simulink model "absolute"  (R2015a)
settings: Solver=ode45  SolverMode=SingleTasking  StartTime=0.0  StopTime=10.0  RelTol=1e-3
model workspace (MAT data in the model file):
  ContractValidatorBlocksMap = containers.Map
  ContractValidatorBlocksMap.serialization.keys = {'absolute/contract/validator'}
  ContractValidatorBlocksMap.serialization.values{1}.block = 'absolute/contract/validator'
  ContractValidatorBlocksMap.serialization.values{1}.assumePorts = 0
  ContractValidatorBlocksMap.serialization.values{1}.guaranteePorts = 2
  ContractValidatorBlocksMap.serialization.values{1}.modeBlocksPorts = 0
  ContractValidatorBlocksMap.serialization.values{1}.portHandles.Inport = [62.0009765625 63.0004882812]
  ContractValidatorBlocksMap.serialization.values{1}.portHandles.Outport = 64.0004882812
  ContractValidatorBlocksMap.serialization.values{1}.portHandles.Enable = []
  ContractValidatorBlocksMap.serialization.values{1}.portHandles.Trigger = []
  ContractValidatorBlocksMap.serialization.values{1}.portHandles.State = []
  ContractValidatorBlocksMap.serialization.values{1}.portHandles.LConn = []
  ContractValidatorBlocksMap.serialization.values{1}.portHandles.RConn = []
  ContractValidatorBlocksMap.serialization.values{1}.portHandles.Ifaction = []
  ContractValidatorBlocksMap.serialization.values{1}.portHandles.Reset = []
  ContractValidatorBlocksMap.serialization.values{1}.portConnectivity(1).Type = '1'
  ContractValidatorBlocksMap.serialization.values{1}.portConnectivity(1).Position = [365 -50]
  ContractValidatorBlocksMap.serialization.values{1}.portConnectivity(1).SrcBlock = 36.0014648438
  ContractValidatorBlocksMap.serialization.values{1}.portConnectivity(1).SrcPort = 0
  ContractValidatorBlocksMap.serialization.values{1}.portConnectivity(1).DstBlock = []
  ContractValidatorBlocksMap.serialization.values{1}.portConnectivity(1).DstPort = []
  ContractValidatorBlocksMap.serialization.values{1}.portConnectivity(2).Type = '2'
  ContractValidatorBlocksMap.serialization.values{1}.portConnectivity(2).Position = [365 200]
  ContractValidatorBlocksMap.serialization.values{1}.portConnectivity(2).SrcBlock = 22.0004882812
  ContractValidatorBlocksMap.serialization.values{1}.portConnectivity(2).SrcPort = 0
  ContractValidatorBlocksMap.serialization.values{1}.portConnectivity(2).DstBlock = []
  ContractValidatorBlocksMap.serialization.values{1}.portConnectivity(2).DstPort = []
  ContractValidatorBlocksMap.serialization.values{1}.portConnectivity(3).Type = '1'
  ContractValidatorBlocksMap.serialization.values{1}.portConnectivity(3).Position = [500 75]
  ContractValidatorBlocksMap.serialization.values{1}.portConnectivity(3).SrcBlock = []
  ContractValidatorBlocksMap.serialization.values{1}.portConnectivity(3).SrcPort = []
  ContractValidatorBlocksMap.serialization.values{1}.portConnectivity(3).DstBlock = 44.0009765625
  ContractValidatorBlocksMap.serialization.values{1}.portConnectivity(3).DstPort = 0
  ContractValidatorBlocksMap.serialization.uniformity = 0
  ContractValidatorBlocksMap.serialization.keyType = 'char'
  ContractValidatorBlocksMap.serialization.valueType = 'any'
undefined symbols (not defined in the file or in its folder): contractAfterSimulation, contractBeforeSimulation, saveValidatorParameters
undefined symbols (not defined in the file): ContractBlock, ContractGuaranteeBlock, ContractValidatorBlock
libraries: simulink x2
settings Model: CovMetricSettings=dwe  CovHtmlReporting=off  covSaveCumulativeToWorkspaceVar=off  CovSaveSingleToWorkspaceVar=off  CovExternalEMLEnable=on  Creator=mahgoubyahia  LastModifiedBy=hbourbou
settings DataIOCC: LimitDataPoints=off  SaveFormat=Dataset
settings DebuggingCC: SFUnexpectedBacktrackingDiag=error  SFNoUnconditionalDefaultTransitionDiag=error
settings HardwareCC: ProdBitPerPointer=64  ProdLargestAtomicFloat=Float  ProdIntDivRoundTo=Zero  ProdEndianess=LittleEndian  ProdHWDeviceType=Specified
settings ModelReferenceCC: PropagateSignalLabelsOutOfModel=on
settings GRTTargetCC: TargetLangStandard=C99 (ISO)  GeneratePreprocessorConditionals=Use local settings

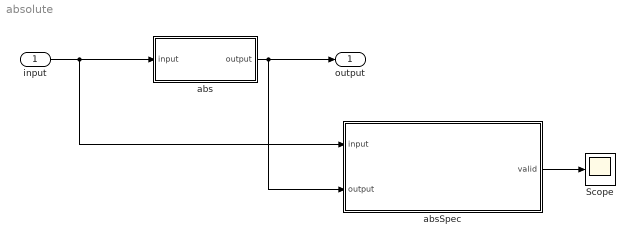
== system absolute ==
  input : Inport  OutDataTypeStr=int32
  Scope : Scope
      settings: TimeRange=auto  MaxDataPoints=5000  SaveToWorkspace=off  SaveName=ScopeData  YMin=-10  YMax=10  SampleTime=-1
  abs : Subsystem
  absSpec : Subsystem  mask{ContractBlockType=ContractBlock}
      mask init:
      | set_param(gcb, 'LinkStatus', 'none');
      mask DialogControl DescTextVar Prompt: Contract block
      mask Display:
      | text(0.5, 0.5, '{\bf\fontsize{20}Contract}', 'hor', 'center', 'texmode','on');
      | blocks = find_system(gcb, 'LookUnderMasks','all', 'SearchDepth',1,'BlockType','Inport');
      | for i = 1 : length(blocks)
      |     blockName = get_param(blocks(i), 'Name');
      |     [path, blockName] = fileparts(char(blockName));
      |     port_label('input', i, blockName);
      | end
      | 
      | blocks = find_system(gcb, 'LookUnderMasks','all', 'SearchDepth',1,'BlockType','Outport');
      | for i = 1 : length(blocks)
      |     blockName = get_param(blocks(i), 'Name');
      |     [path, blockName] = fileparts(char(blockName));
      |     port_label('output', i, blockName);
      | end
  output : Outport
  wires:
  input/1 -> absSpec/1(input), abs/1(input)
  absSpec/1(valid) -> Scope/1
  abs/1(output) -> absSpec/2(output), output/1

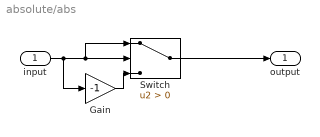
== system absolute/abs ==
  input : Inport
  Gain : Gain  Gain=-1  OutDataTypeStr=int32
  Switch : Switch  Criteria=u2 > Threshold
  output : Outport
  wires:
  Switch/1 -> output/1
  input/1 -> Gain/1, Switch/1, Switch/2
  Gain/1 -> Switch/3

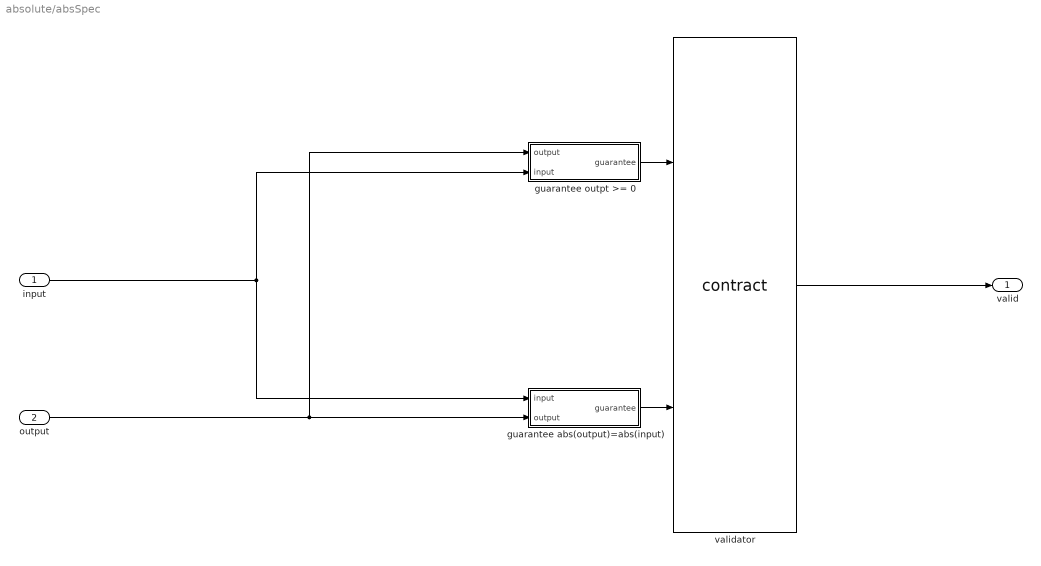
== system absolute/absSpec ==
  input : Inport  OutDataTypeStr=int32
  output : Inport  Port=2  OutDataTypeStr=int32
  guarantee abs(output)=abs(input) : Subsystem  mask{ContractBlockType=ContractGuaranteeBlock}
      mask init:
      | set_param(gcb, 'LinkStatus', 'none');
      mask DialogControl DescTextVar Prompt: Guarantee block
  guarantee outpt >= 0 : Subsystem  mask{ContractBlockType=ContractGuaranteeBlock}
      mask init:
      | set_param(gcb, 'LinkStatus', 'none');
      mask DialogControl DescTextVar Prompt: Guarantee block
  validator : M-S-Function  LoadFcn=saveValidatorParameters(gcb);  InitFcn=contractBeforeSimulation();  StopFcn=contractAfterSimulation();  FunctionName=contract  mask(KindContractValidator){assumePorts=0, guaranteePorts=2, modePorts=0, ContractBlockType=ContractValidatorBlock, createInportsCheckbox=on}
      mask prompts: assumePorts "Assume ports     :"; guaranteePorts "Guarantee ports :"; modePorts "Mode ports        :"; createInportsCheckbox "Create inports and connect them automatically"
      mask init:
      | set_param(gcb,'LinkStatus','none');
      | contract_callback('inputs_callback',gcb);
      mask DialogControl DescTextVar Prompt: The validator block implements the following logic: <br> <br> <b>Sofar</b>(assume<sub>1</sub> <b>&#8743;</b> assume<sub>2</sub> <b>&#8743;</b> ... assume<sub>k</sub>) <b>&rarr;</b> (guarantee<sub>1</sub> <b>&#8743;</b> guarantee<sub>2</sub> <b>&#8743;</b> ... guarantee<sub>m</sub> <b>&#8743;</b>  mode<sub>1</sub> <b>&#8743;</b> mode<sub>2</sub> <b>&#8743;</b> ... <b>&#8743;</b> mode<sub>n</sub> )<br> where mode<sub>i</sub> = require<sub>i</sub> <b>&rarr;</b> ensure<sub>i</sub>
      mask Display:
      | color('black');
      | port_label('input',1,'guarantee');
      | port_label('input',2,'guarantee');
      | port_label('output',1,'valid');
  valid : Outport
  wires:
  validator/1 -> valid/1
  input/1 -> guarantee abs(output)=abs(input)/1(input), guarantee outpt >= 0/2(input)
  output/1 -> guarantee abs(output)=abs(input)/2(output), guarantee outpt >= 0/1(output)
  guarantee abs(output)=abs(input)/1(guarantee) -> validator/2
  guarantee outpt >= 0/1(guarantee) -> validator/1

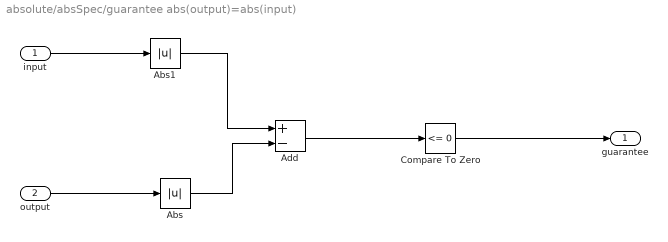
== system absolute/absSpec/guarantee abs(output)=abs(input) ==
  input : Inport
  output : Inport  Port=2
  Abs : Abs
  Abs1 : Abs
  Add : Sum  Inputs=+-
  Compare To Zero : simulink/Logic and Bit Operations/Compare To Zero  relop=<=  OutDataTypeStr=boolean
  guarantee : Outport  OutDataTypeStr=boolean
  wires:
  output/1 -> Abs/1
  input/1 -> Abs1/1
  Abs1/1 -> Add/1
  Abs/1 -> Add/2
  Add/1 -> Compare To Zero/1
  Compare To Zero/1 -> guarantee/1

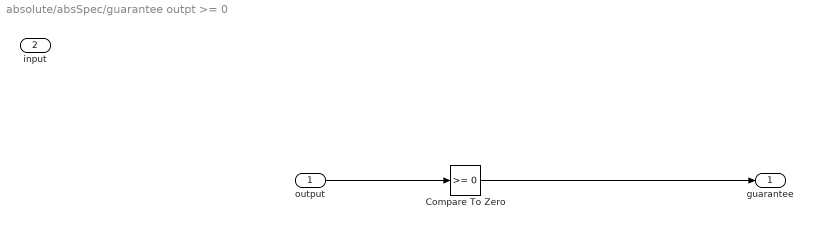
== system absolute/absSpec/guarantee outpt >= 0 ==
  output : Inport
  input : Inport  Port=2
  Compare To Zero : simulink/Logic and Bit Operations/Compare To Zero  relop=>=  OutDataTypeStr=boolean
  guarantee : Outport  OutDataTypeStr=boolean
  wires:
  output/1 -> Compare To Zero/1
  Compare To Zero/1 -> guarantee/1
